simulink model "accel_sim"  (Simulink 8.8)
settings: Solver=FixedStepDiscrete  StartTime=0.0  StopTime=10.0  RelTol=1e-3
libraries: sphero_lib x5
settings Model: Creator=gcampa  LastModifiedBy=gcampa
settings DataIOCC: SignalLoggingSaveFormat=Dataset
settings OptimizationCC: BlockReduction=off  BooleanDataType=off
settings DebuggingCC: SaveWithParameterizedLinksMsg=none  SignalResolutionControl=TryResolveAllWithWarning  FcnCallInpInsideContextMsg=error  StateNameClashWarn=none
settings HardwareCC: TargetUnknown=on
settings GRTTargetCC: CombineOutputUpdateFcns=on  GRTInterface=off

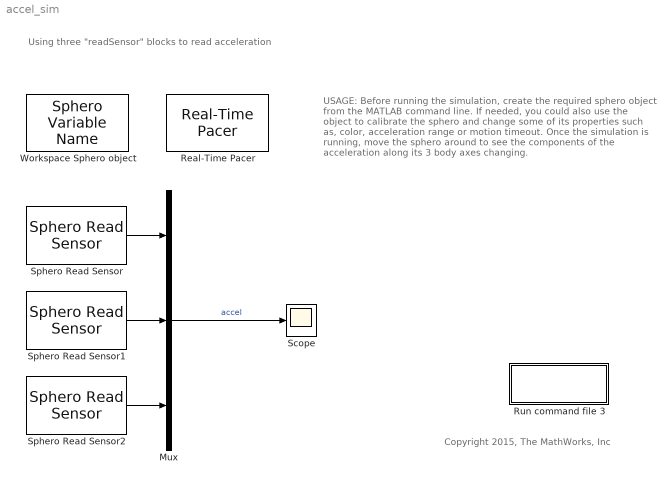
== system accel_sim ==
  note: Copyright 2015, The MathWorks, Inc
  note: USAGE:
      |
      | Before running the simulation, create the required sphero object
      | from the MATLAB command line. If needed, you could also use
      | the object to calibrate the sphero and change some of its properties
      | such as, color, acceleration range or motion timeout.
      |
      | Once the simulation is running, move the sphero around to see the
      | components of the acceleration along its 3 body axes changing.
  note: Using three "readSensor" blocks to read acceleration
  Mux : Mux  Inputs=3
  Real-Time Pacer : sphero_lib/Real-Time Pacer  simTimePerRealTime=1
  Run command file 3 : Subsystem
      settings: OpenFcn=sphero_lib
      mask Display: disp('Open Main\nSimulink Library')
  Scope : Scope
  Sphero Read Sensor : sphero_lib/Sphero Read Sensor  SpheroVarNumber=Existing workspace Sphero variable #1  SensorString=accelX  T=0.1
  Sphero Read Sensor1 : sphero_lib/Sphero Read Sensor  SpheroVarNumber=Existing workspace Sphero variable #1  SensorString=accelY  T=0.1
  Sphero Read Sensor2 : sphero_lib/Sphero Read Sensor  SpheroVarNumber=Existing workspace Sphero variable #1  SensorString=accelZ  T=0.1
  Workspace Sphero object : sphero_lib/Sphero Variable Name  Priority=3  SpheroVarNumber=Existing workspace Sphero variable #1  workspaceVarName=sph
  wires:
  Mux/1 -> Scope/1  "accel"
  Sphero Read Sensor2/1 -> Mux/3
  Sphero Read Sensor/1 -> Mux/1
  Sphero Read Sensor1/1 -> Mux/2

== system accel_sim/Run command file 3 ==
